simulink model "aufgabe1_linear_anfangsbedingung1"  (R2023b)
settings: Solver=FixedStepAuto  StartTime=0.0  StopTime=10.0  FixedStep=0.001  RelTol=1e-3
settings Model: Creator=serkan  LastModifiedBy=serkan

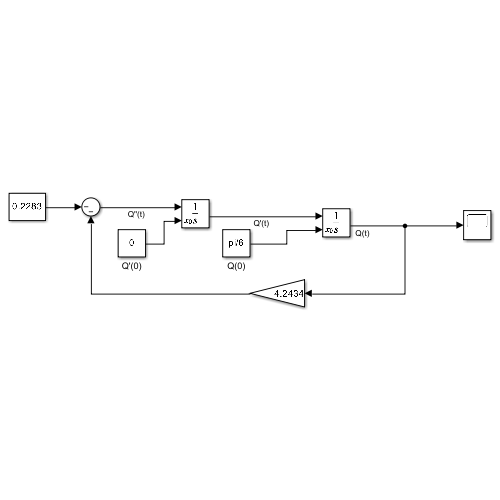
[thumbnail: Simulink's stored preview of the top-level diagram]
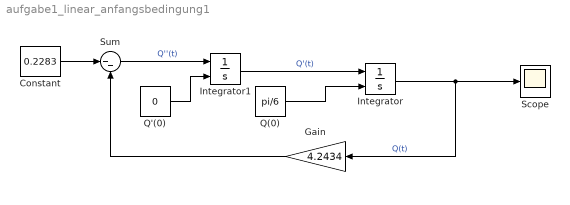
== system aufgabe1_linear_anfangsbedingung1 ==
  Constant : Constant  Value=0.2283
  Gain : Gain  Gain=4.2434
  Integrator : Integrator  InitialConditionSource=external  InitialCondition=pi/6
  Integrator1 : Integrator  InitialConditionSource=external
  Q'(0) : Constant  Value=0
  Q(0) : Constant  Value=pi/6
  Scope : Scope
  Sum : Sum  Inputs=|--
  wires:
  Integrator/1 -> Scope/1, Gain/1  "Q(t)"
  Integrator1/1 -> Integrator/1  "Q'(t)"
  Gain/1 -> Sum/2
  Sum/1 -> Integrator1/1  "Q''(t)"
  Q(0)/1 -> Integrator/2
  Constant/1 -> Sum/1
  Q'(0)/1 -> Integrator1/2
